simulink model "solar_collector_hot_water_tank"  (R2017a)
settings: Solver=VariableStepAuto  StartTime=0.0  StopTime=100000  RelTol=1e-3
values from neighbouring files (symbols this model uses):
  a1 = Ac*eta/C_c    (= 0.000575964912281)    [Linearized_model.m]    (also in Linearized_model_v1.m; Maple_linearization.m = 0.000380952380952; solar_collector_init.m = 7.33988724098e-05)
  a2 = -U_L1*Ac/2/C_c    (= -0.00145487240829)    [Linearized_model.m]    (also in Linearized_model_v1.m = -0.00290974481659; Maple_linearization.m = 0.00111111111111; solar_collector_init.m = -0.000214080044529)
  a3 = -U_L2*Ac/C_c    (= -7.48006379585e-06)    [Linearized_model.m]    (also in Linearized_model_v1.m; Maple_linearization.m = -0.00222222222222; solar_collector_init.m = 0.000428160089057)
  a4 = V_c^-1    (= 333.333333333)    [Linearized_model.m]    (also in Linearized_model_v1.m; Maple_linearization.m = 666.666666667; solar_collector_init.m = 133.333333333)
  a5 = -a4    (= -333.333333333)    [Linearized_model.m]    (also in Linearized_model_v1.m; Maple_linearization.m = -666.666666667; solar_collector_init.m = -133.333333333)
libraries: simulink x1
settings Model: Creator=info  LastModifiedBy=admin

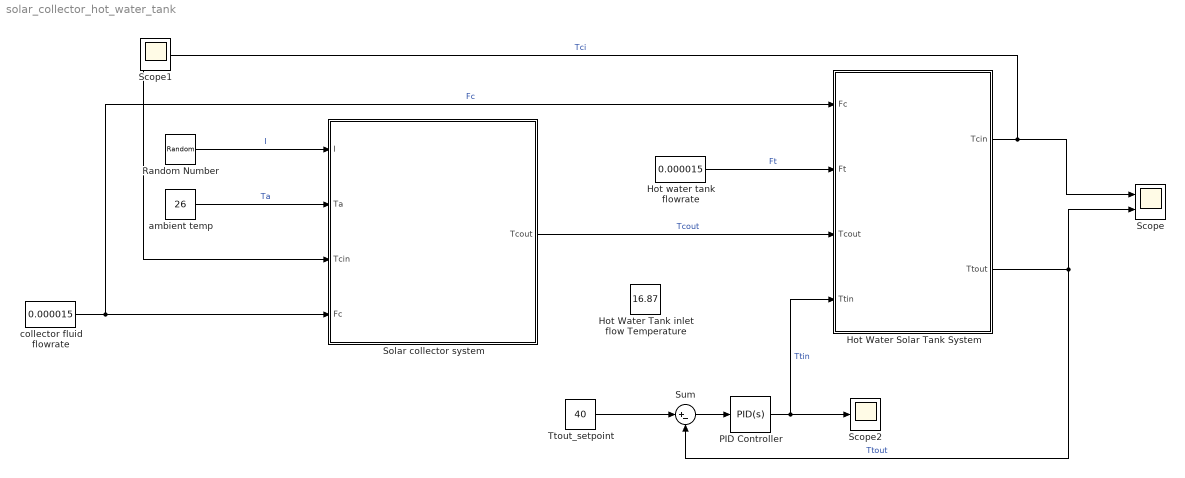
== system solar_collector_hot_water_tank ==
  Hot Water Solar Tank System : Subsystem
      mask Display: image('storage_tank.PNG');
  Hot Water Tank inlet flow Temperature : Constant  Value=16.87
  Hot water tank flowrate : Constant  Value=0.000015
  PID Controller : simulink/Continuous/PID Controller  Controller=PID  TimeDomain=Continuous-time  SampleTime=-1  IntegratorMethod=Forward Euler  FilterMethod=Forward Euler  Form=Parallel  UseFilter=on  ControllerParametersSource=internal  P=1.1  I=0.0005  D=0.001  N=100  InitialConditionSource=internal  InitialConditionForIntegrator=0  InitialConditionForFilter=0  ExternalReset=none  LimitOutput=on  UpperSaturationLimit=35  LowerSaturationLimit=0  LinearizeAsGain=on  AntiWindupMode=none  Kb=1  TrackingMode=off  Kt=1  PParamMin=[]  PParamMax=[]  IParamMin=[]  IParamMax=[]  DParamMin=[]  DParamMax=[]  NParamMin=[]  NParamMax=[]  KbParamMin=[]  KbParamMax=[]  KtParamMin=[]  KtParamMax=[]  POutMin=[]  POutMax=[]  IOutMin=[]  IOutMax=[]  DOutMin=[]  DOutMax=[]  NOutMin=[]  NOutMax=[]  KbOutMin=[]  KbOutMax=[]  KtOutMin=[]  KtOutMax=[]  IntegratorOutMin=[]  IntegratorOutMax=[]  FilterOutMin=[]  FilterOutMax=[]  SumOutMin=[]  SumOutMax=[]  SumI1OutMin=[]  SumI1OutMax=[]  SumI2OutMin=[]  SumI2OutMax=[]  SumI3OutMin=[]  SumI3OutMax=[]  SumDOutMin=[]  SumDOutMax=[]  SaturationOutMin=[]  SaturationOutMax=[]  IntegratorContinuousStateAttributes=''  IntegratorStateMustResolveToSignalObject=off  IntegratorRTWStateStorageClass=Auto  FilterContinuousStateAttributes=''  FilterStateMustResolveToSignalObject=off  FilterRTWStateStorageClass=Auto  DifferentiatorICPrevScaledInput=0  DifferentiatorOutMin=[]  DifferentiatorOutMax=[]  InitialConditionSetting=State (most efficient)
  Random Number : RandomNumber  Mean=1360  Variance=0.5  SampleTime=0.1
  Scope : Scope  NumInputPorts=2
  Scope2 : Scope
  Solar collector system : Subsystem
      mask Display: image('collector_image.jpg');
  Sum : Sum  Inputs=|+-
  Ttout_setpoint : Constant  Value=40
  ambient temp : Constant  Value=26
  collector fluid flowrate : Constant  Value=0.000015
  Scope1 : Scope
  wires:
  Solar collector system/1(Tcout) -> Hot Water Solar Tank System/3("Tcout ")  "Tcout"
  Hot Water Solar Tank System/1("Tcin ") -> Solar collector system/3(Tcin), Scope/1  "Tci"
  ambient temp/1 -> Solar collector system/2(Ta)  "Ta"
  Random Number/1 -> Solar collector system/1(I)  "I"
  PID Controller/1 -> Hot Water Solar Tank System/4("Ttin "), Scope2/1  "Ttin"
  Hot Water Solar Tank System/2("Ttout ") -> Sum/2, Scope/2  "Ttout"
  Ttout_setpoint/1 -> Sum/1
  Sum/1 -> PID Controller/1
  collector fluid flowrate/1 -> Hot Water Solar Tank System/1("Fc "), Solar collector system/4(Fc)  "Fc"
  Hot water tank flowrate/1 -> Hot Water Solar Tank System/2(Ft)  "Ft"

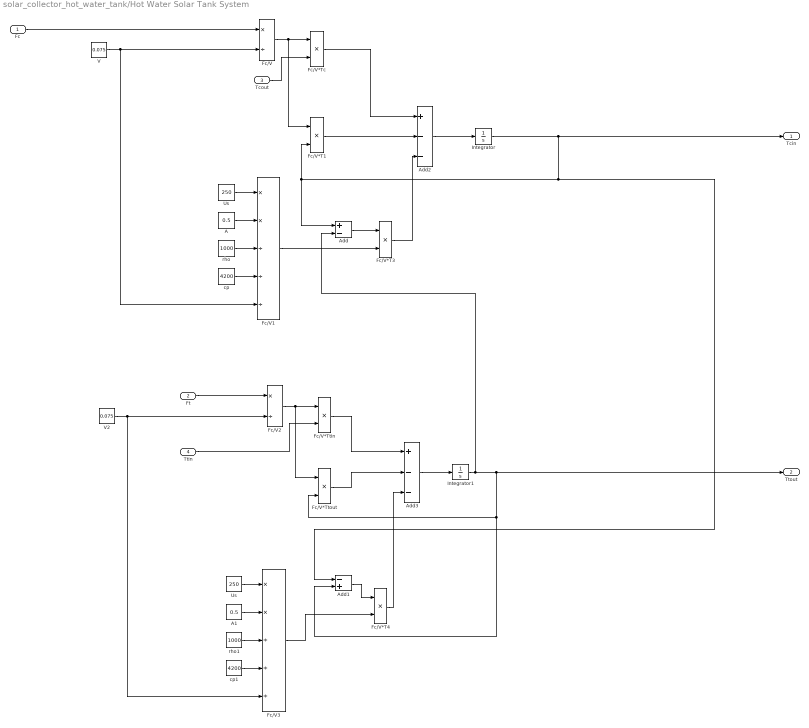
== system solar_collector_hot_water_tank/Hot Water Solar Tank System ==
  "Fc " : Inport
  Ft : Inport  Port=2
  "Tcout " : Inport  Port=3
  "Ttin " : Inport  Port=4
  A : Constant  Value=0.5
  A1 : Constant  Value=0.5
  Add : Sum  Inputs=+-
  Add1 : Sum  Inputs=-+
  Add2 : Sum  Inputs=+--
  Add3 : Sum  Inputs=+--
  Fc/V : Product  Inputs=*/
  Fc/V*T1 : Product  Inputs=**
  Fc/V*T3 : Product  Inputs=**
  Fc/V*T4 : Product  Inputs=**
  Fc/V*Tc : Product  Inputs=**
  Fc/V*Ttin : Product  Inputs=**
  Fc/V*Ttout : Product  Inputs=**
  Fc/V1 : Product  Inputs=**///
  Fc/V2 : Product  Inputs=*/
  Fc/V3 : Product  Inputs=**///
  Integrator : Integrator  InitialCondition=16.87
  Integrator1 : Integrator  InitialCondition=10
  Us : Constant  Value=250
  "Us    " : Constant  Value=250
  V : Constant  Value=0.075
  V2 : Constant  Value=0.075
  cp : Constant  Value=4200
  cp1 : Constant  Value=4200
  rho : Constant  Value=1000
  rho1 : Constant  Value=1000
  "Tcin " : Outport
  "Ttout " : Outport  Port=2
  wires:
  V/1 -> Fc/V1/5, Fc/V/2
  "Us    "/1 -> Fc/V3/1
  Integrator1/1 -> Add1/2, Fc/V*Ttout/2, "Ttout "/1, Add/2
  "Ttin "/1 -> Fc/V*Ttin/2
  "Fc "/1 -> Fc/V/1
  Fc/V/1 -> Fc/V*T1/1, Fc/V*Tc/1
  rho/1 -> Fc/V1/3
  cp1/1 -> Fc/V3/4
  A1/1 -> Fc/V3/2
  Integrator/1 -> "Tcin "/1, Add1/1, Fc/V*T1/2, Add/1
  Us/1 -> Fc/V1/1
  "Tcout "/1 -> Fc/V*Tc/2
  rho1/1 -> Fc/V3/3
  Fc/V2/1 -> Fc/V*Ttin/1, Fc/V*Ttout/1
  V2/1 -> Fc/V2/2, Fc/V3/5
  Ft/1 -> Fc/V2/1
  cp/1 -> Fc/V1/4
  A/1 -> Fc/V1/2
  Fc/V*Tc/1 -> Add2/1
  Add2/1 -> Integrator/1
  Fc/V1/1 -> Fc/V*T3/2
  Fc/V*T3/1 -> Add2/3
  Fc/V*Ttin/1 -> Add3/1
  Add3/1 -> Integrator1/1
  Add/1 -> Fc/V*T3/1
  Fc/V*T1/1 -> Add2/2
  Fc/V*Ttout/1 -> Add3/2
  Fc/V*T4/1 -> Add3/3
  Fc/V3/1 -> Fc/V*T4/2
  Add1/1 -> Fc/V*T4/1

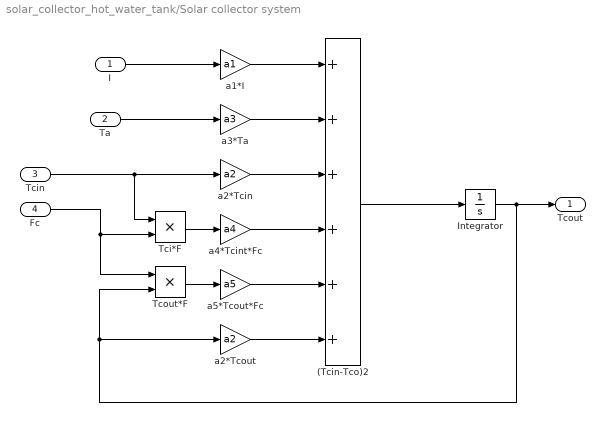
== system solar_collector_hot_water_tank/Solar collector system ==
  I : Inport
  Ta : Inport  Port=2
  Tcin : Inport  Port=3
  Fc : Inport  Port=4
  (Tcin-Tco)2 : Sum  Inputs=++++++
  Integrator : Integrator  InitialCondition=10
  Tci*F : Product  Inputs=**
  Tcout*F : Product  Inputs=**
  a1*I : Gain  Gain=a1
  a2*Tcin : Gain  Gain=a2
  "a2*Tcout " : Gain  Gain=a2
  a3*Ta : Gain  Gain=a3
  a4*Tcint*Fc : Gain  Gain=a4
  "a5*Tcout*Fc " : Gain  Gain=a5
  Tcout : Outport
  wires:
  I/1 -> a1*I/1
  Integrator/1 -> "a2*Tcout "/1, Tcout*F/2, Tcout/1
  (Tcin-Tco)2/1 -> Integrator/1
  Fc/1 -> Tcout*F/1, Tci*F/2
  a1*I/1 -> (Tcin-Tco)2/1
  Ta/1 -> a3*Ta/1
  Tcin/1 -> Tci*F/1, a2*Tcin/1
  a3*Ta/1 -> (Tcin-Tco)2/2
  a2*Tcin/1 -> (Tcin-Tco)2/3
  "a5*Tcout*Fc "/1 -> (Tcin-Tco)2/5
  Tci*F/1 -> a4*Tcint*Fc/1
  a4*Tcint*Fc/1 -> (Tcin-Tco)2/4
  Tcout*F/1 -> "a5*Tcout*Fc "/1
  "a2*Tcout "/1 -> (Tcin-Tco)2/6
